simulink model "Intergration_ACC"  (R2018b)
(part 3 of 31)

  EPS_HSC2_FrP03_0x1EC/1 -> Data Type Conversion64/1  "ChLKACtrlStsHSC2"
  EPS_HSC2_FrP03_0x1EC/2 -> Data Type Conversion65/1  "DrvrStrgDlvrdToqVHSC2"
  EPS_HSC2_FrP03_0x1EC/3 -> Data Type Conversion66/1  "DrvrStrgDlvrdToqHSC2"
  EPS_HSC2_FrP03_0x1EC/5 -> Data Type Conversion67/1  "ChLKARespToqHSC2"
  EPS_HSC2_FrP03_0x1EC/6 -> Data Type Conversion68/1  "ChLKARespToqVHSC2"
  SCS_HSC2_FrP24_0x251/2 -> Data Type Conversion69/1  "VehTrgtLongtAccHSC2"
  Data Type Conversion69/1 -> Bus Creator16/1
  Data Type Conversion70/1 -> Bus Creator16/2
  SCS_HSC2_FrP24_0x251/4 -> Data Type Conversion70/1  "ChAEBDclReqRespHSC2"
  Data Type Conversion71/1 -> Bus Creator16/3
  SCS_HSC2_FrP24_0x251/5 -> Data Type Conversion71/1  "ChACCAEBBrkJerkReqRespHSC2"
  Data Type Conversion72/1 -> Bus Creator16/4
  SCS_HSC2_FrP24_0x251/6 -> Data Type Conversion72/1  "ChAEBPrflReqRespHSC2"
  Data Type Conversion73/1 -> Bus Creator16/5
  SCS_HSC2_FrP24_0x251/7 -> Data Type Conversion73/1  "ChACCReqFlrStsHSC2"
  Data Type Conversion74/1 -> Bus Creator16/6
  SCS_HSC2_FrP24_0x251/8 -> Data Type Conversion74/1  "ChAEBHydBrkAstReqRespHSC2"
  Data Type Conversion75/1 -> Bus Creator16/7
  SCS_HSC2_FrP24_0x251/9 -> Data Type Conversion75/1  "ChACCAccReqRespHSC2"
  Data Type Conversion76/1 -> Bus Creator16/8
  SCS_HSC2_FrP24_0x251/10 -> Data Type Conversion76/1  "VehSdslStsHSC2"
  Data Type Conversion77/1 -> Bus Creator17/1
  GW_HSC2_HCU_FrP13_0x19C/2 -> Data Type Conversion77/1  "EPTTrInptShaftSpdHSC2"
  Data Type Conversion78/1 -> Bus Creator17/2
  GW_HSC2_HCU_FrP13_0x19C/3 -> Data Type Conversion78/1  "EPTTrInptShaftToqHSC2"
  Data Type Conversion79/1 -> Bus Creator17/3
  GW_HSC2_HCU_FrP13_0x19C/4 -> Data Type Conversion79/1  "EPTTrInptShaftSpdVHSC2"
  Data Type Conversion80/1 -> Bus Creator17/4
  GW_HSC2_HCU_FrP13_0x19C/5 -> Data Type Conversion80/1  "EPTTrInptShaftToqVHSC2"
  Bus Creator17/1 -> Bus Creator9/17
  Bus Creator16/1 -> Bus Creator9/16
